simulink model "ClosedLoop_FFL"  (R2022b)
settings: Solver=VariableStepAuto  StartTime=0.0  StopTime=T_end  RelTol=1e-3
settings Model: Creator=andras  LastModifiedBy=andras

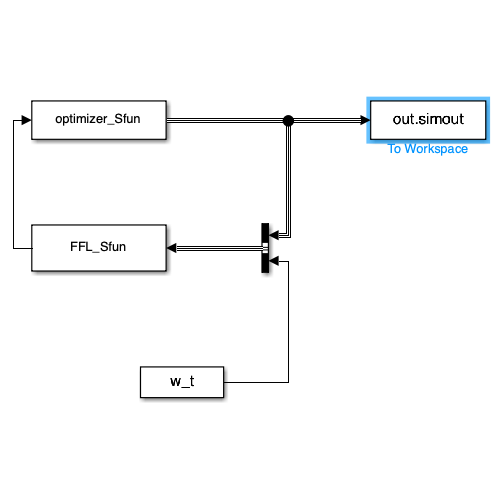
[thumbnail: Simulink's stored preview of the top-level diagram]
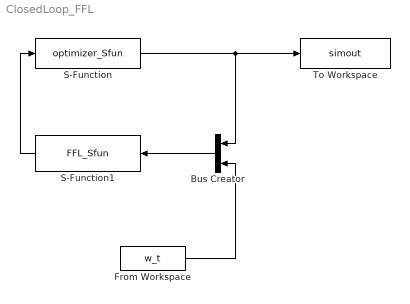
== system ClosedLoop_FFL ==
  Bus Creator : BusCreator  Inputs=2
  From Workspace : FromWorkspace  VariableName=w_t
  S-Function : S-Function  FunctionName=optimizer_Sfun  SFunctionDeploymentMode=off  EnableBusSupport=off
  S-Function1 : S-Function  FunctionName=FFL_Sfun  SFunctionDeploymentMode=off  EnableBusSupport=off
  To Workspace : ToWorkspace  VariableName=simout  SaveFormat=Timeseries  SampleTime=-1
  wires:
  S-Function1/1 -> S-Function/1
  Bus Creator/1 -> S-Function1/1
  From Workspace/1 -> Bus Creator/2
  S-Function/1 -> To Workspace/1, Bus Creator/1
